simulink model "automotiveSystems_termp"  (R2020a)
settings: Solver=VariableStepAuto  StartTime=0.0  StopTime=30  MaxStep=1e-2  RelTol=1e-3  AbsTol=1e-3  EnableMultiTasking=on
PreLoadFcn:
  | GeRa.Ct = 1.384;
  | GeRa.G1 = 2.5918;
  | GeRa.G2 = 1.4601;
  | GeRa.G3 = 1;
undefined symbols (not defined in the file): sigbuilder_block
libraries: fl_lib x53, sdl_lib x20, nesl_utility x12, fl_ps_legacy_lib x11, eeGeneralControl x1, autolibsharedtransfixedgear x1
(part 2 of 4)

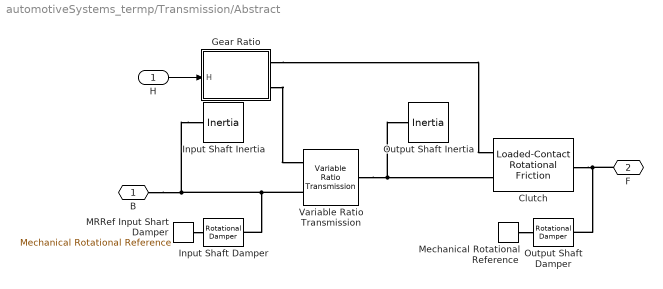
== system automotiveSystems_termp/Transmission/Abstract ==
  H : Inport
  Clutch : sdl_lib/Brakes & Detents/Rotational/Loaded-Contact Rotational Friction  geometry_model=1  r_eff=300 mm  d_o=150 mm  d_i=100 mm  friction_model=1  mu_w_vector=[ 0 0.1 0.2 0.3 0.4 0.5 1 2 5 10 100 1000 ] rad/s  temperature_TLU=[280.0, 300.0, 320.0] K  mu_static=0.5  mu_static_vector=[0.4, 0.38, 0.36]  mu_coulomb=0.46  mu_coulomb_vector=[ 0.29 0.28 0.26 0.22 0.21 0.2 0.2 0.19 0.19 0.19 0.19 0.19 ]  mu_coulomb_temp_vector=[0.3, 0.28, 0.25]  mu_coulomb_matrix=[0.34, 0.32, 0.3; 0.3, 0.28, 0.25; 0.25, 0.2, 0.15]  mu_interp_method=1  mu_extrap_method=1  w_tol=0.001 rad/s  force_min=100 N  mu_visc=0 N*m/(rad/s)  initial_state_locked=0  thermal_mass=50 kJ/K  T_init=300 K
      settings: SourceProductBaseCode=LD  InternalSimscapePortConfiguration="{\"Bottom\":[],\"Left\":[{\"id\":\"N\",\"label\":\"N\",\"type\":\"input\"},{\"id\":\"B\",\"label\":\"B\",\"type\":\"foundation.mechanical.rotational.rotational\"}],\"Right\":[{\"id\":\"F\",\"label\":\"F\",\"type\":\"foundation.mechanical.rotational.rotational\"}],\"Top\":[]}"
  Gear Ratio : Subsystem
  Input Shaft Damper : fl_lib/Mechanical/Rotational Elements/Rotational Damper  D=0.01*10 N*m/(rad/s)  w_specify=off  w_priority=High  w=0 rad/s  w_nominal_specify=off  w_nominal_unit=rad/s  w_nominal_value=1  t_specify=off  t_priority=High  t=0 N*m  t_nominal_specify=off  t_nominal_unit=N*m  t_nominal_value=1
  Input Shaft Inertia : fl_lib/Mechanical/Rotational Elements/Inertia  inertia=0.026 kg*m^2  w_specify=off  w_priority=High  w=0 rad/s  w_nominal_specify=off  w_nominal_unit=rad/s  w_nominal_value=1  t_specify=off  t_priority=High  t=0 N*m  t_nominal_specify=off  t_nominal_unit=N*m  t_nominal_value=1
  MRRef Input Shart Damper : fl_lib/Mechanical/Rotational Elements/Mechanical Rotational Reference
  Mechanical Rotational Reference : fl_lib/Mechanical/Rotational Elements/Mechanical Rotational Reference
  Output Shaft Damper : fl_lib/Mechanical/Rotational Elements/Rotational Damper  D=0.01 N*m/(rad/s)  w_specify=off  w_priority=High  w=0 rad/s  w_nominal_specify=off  w_nominal_unit=rad/s  w_nominal_value=1  t_specify=off  t_priority=High  t=0 N*m  t_nominal_specify=off  t_nominal_unit=N*m  t_nominal_value=1
  Output Shaft Inertia : fl_lib/Mechanical/Rotational Elements/Inertia  inertia=0.034 kg*m^2  w_specify=on  w_priority=High  w=0 rad/s  w_nominal_specify=off  w_nominal_unit=rad/s  w_nominal_value=1  t_specify=off  t_priority=High  t=0 N*m  t_nominal_specify=off  t_nominal_unit=N*m  t_nominal_value=1
  Variable Ratio Transmission : sdl_lib/Couplings & Drives/Variable Ratio Transmission  rotation_direction=1  kp=1e+5 N*m/rad  kv=10 N*m/(rad/s)  initial_torque=0 N*m  losses_model=1  efficiency=0.85  mu_visc=[ 0 0 ] N*m/(rad/s)  w_thr=0.01 rad/s  R_specify=off  R_priority=None  R=1  R_nominal_specify=off  R_nominal_unit=1  R_nominal_value=1
      settings: SourceProductBaseCode=LD  InternalSimscapePortConfiguration="{\"Bottom\":[],\"Left\":[{\"id\":\"ratio\",\"label\":\"r\",\"type\":\"input\"},{\"id\":\"B\",\"label\":\"B\",\"type\":\"foundation.mechanical.rotational.rotational\"}],\"Right\":[{\"id\":\"F\",\"label\":\"F\",\"type\":\"foundation.mechanical.rotational.rotational\"}],\"Top\":[]}"
  B : PMIOPort  Side=Left
  F : PMIOPort  Port=2  Side=Right
  wires:
  H/1 -> Gear Ratio/1(H)
  connections:
  F/RConn1 -- Clutch/RConn1 -- Output Shaft Damper/LConn1
  MRRef Input Shart Damper/LConn1 -- Input Shaft Damper/RConn1
  Mechanical Rotational Reference/LConn1 -- Output Shaft Damper/RConn1
  Input Shaft Inertia/LConn1 -- Variable Ratio Transmission/LConn2 -- Input Shaft Damper/LConn1 -- B/RConn1
  Variable Ratio Transmission/RConn1 -- Clutch/LConn2 -- Output Shaft Inertia/LConn1
  Gear Ratio/RConn2 -- Variable Ratio Transmission/LConn1
  Gear Ratio/RConn1 -- Clutch/LConn1
